simulink model "MdInOutChk"  (R2018b)
settings: Solver=FixedStepDiscrete  StartTime=0.0  StopTime=10.0  FixedStep=0.01  RelTol=1e-3
undefined symbols (not defined in the file or in its folder): MdRspLocal2
libraries: OutRspChkLib x20
(part 2 of 2)

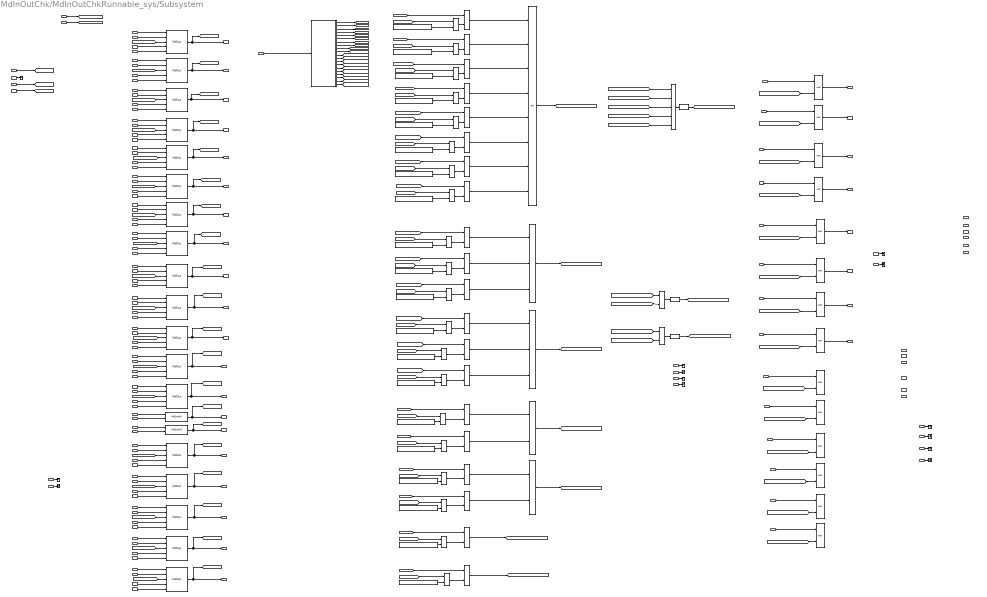
== system MdInOutChk/MdInOutChkRunnable_sys/Subsystem ==
  acsEntyMdReq_Val_read : Inport
  acsExtMdReq_Val_read : Inport  Port=2
  AllLugMdReq_Val_read : Inport  Port=3
  AllVipMdReq_Val_read : Inport  Port=4
  CommExitCond_Val_read : Inport  Port=5
  CommExitCondwithSpeed_Val_read : Inport  Port=6
  IntimacyRtMdReq_Val_read : Inport  Port=7
  INTMMdReq_Val_read : Inport  Port=8
  isAcsMdEntryDoneFailed_Val_read : Inport  Port=9
  isAcsMdEntryDoneOK_Val_read : Inport  Port=10
  isAcsMdExtDoneFailed_Val_read : Inport  Port=11
  isAcsMdExtDoneOK_Val_read : Inport  Port=12
  isINTMDoneFailed_Val_read : Inport  Port=13
  isINTMDoneOK_Val_read : Inport  Port=14
  isINTMRDoneFailed_Val_read : Inport  Port=15
  isINTMRDoneOK_Val_read : Inport  Port=16
  isLfFamlyDoneFailed_Val_read : Inport  Port=17
  isLfFamlyDoneOK_Val_read : Inport  Port=18
  isLfLugDoneFailed_Val_read : Inport  Port=19
  isLfLugDoneOK_Val_read : Inport  Port=20
  isLfLyDoneFailed_Val_read : Inport  Port=21
  isLfLyDoneOK_Val_read : Inport  Port=22
  isLfRecoveryDoneFailed_Val_read : Inport  Port=23
  isLfRecoveryDoneOK_Val_read : Inport  Port=24
  isLfVipDoneFailed_Val_read : Inport  Port=25
  isLfVipDoneOK_Val_read : Inport  Port=26
  isLgrstCloseLDoneFailed_Val_read : Inport  Port=27
  isLgrstCloseLDoneOK_Val_read : Inport  Port=28
  isLgrstCloseRDoneFailed_Val_read : Inport  Port=29
  isLgrstCloseRDoneOK_Val_read : Inport  Port=30
  isLgrstOpenLDoneFailed_Val_read : Inport  Port=31
  isLgrstOpenLDoneOK_Val_read : Inport  Port=32
  isLgrstOpenRDoneFailed_Val_read : Inport  Port=33
  isLgrstOpenRDoneOK_Val_read : Inport  Port=34
  isRfFamlyDoneFailed_Val_read : Inport  Port=35
  isRfFamlyDoneOK_Val_read : Inport  Port=36
  isRtLugDoneFailed_Val_read : Inport  Port=37
  isRtLugDoneOK_Val_read : Inport  Port=38
  isRtLyDoneFailed_Val_read : Inport  Port=39
  isRtLyDoneOK_Val_read : Inport  Port=40
  isRtRecoveryDoneFailed_Val_read : Inport  Port=41
  isRtRecoveryDoneOK_Val_read : Inport  Port=42
  isRtVipDoneFailed_Val_read : Inport  Port=43
  isRtVipDoneOK_Val_read : Inport  Port=44
  LfFamlyReq_Val_read : Inport  Port=45
  LfLyMdReq_Val_read : Inport  Port=46
  LgrstCloseLtMdReq_Val_read : Inport  Port=47
  LgrstCloseRtMdReq_Val_read : Inport  Port=48
  LgrstOpenLtMdReq_Val_read : Inport  Port=49
  LgrstOpenRtMdReq_Val_read : Inport  Port=50
  LtLugMdReq_Val_read : Inport  Port=51
  LtRcvyMdReq_Val_read : Inport  Port=52
  LtVipMdReq_Val_read : Inport  Port=53
  LugMdLtAvl_Val_read : Inport  Port=54
  LugMdRtAvl_Val_read : Inport  Port=55
  R3LMdSeatOccupied_Val_read : Inport  Port=56
  R3RMdSeatOccupied_Val_read : Inport  Port=57
  RtFamlyMdReq_Val_read : Inport  Port=58
  RtLugMdReq_Val_read : Inport  Port=59
  RtLyMdReq_Val_read : Inport  Port=60
  RtRcvyMdReq_Val_read : Inport  Port=61
  RtVipMdReq_Val_read : Inport  Port=62
  SoftIntAcsEnty_Val_read : Inport  Port=63
  SoftIntAcsExt_Val_read : Inport  Port=64
  SoftIntAllLug_Val_read : Inport  Port=65
  SoftIntAllVip_Val_read : Inport  Port=66
  SoftIntIntimacyRt_Val_read : Inport  Port=67
  SoftIntINTM_Val_read : Inport  Port=68
  SoftIntLfFamly_Val_read : Inport  Port=69
  SoftIntLfLug_Val_read : Inport  Port=70
  SoftIntLfLy_Val_read : Inport  Port=71
  SoftIntLfRcvy_Val_read : Inport  Port=72
  SoftIntLfVip_Val_read : Inport  Port=73
  SoftIntLgrstCloseLt_Val_read : Inport  Port=74
  SoftIntLgrstCloseRt_Val_read : Inport  Port=75
  SoftIntLgrstOpenLt_Val_read : Inport  Port=76
  SoftIntLgrstOpenRt_Val_read : Inport  Port=77
  SoftIntRtFamly_Val_read : Inport  Port=78
  SoftIntRtLug_Val_read : Inport  Port=79
  SoftIntRtLy_Val_read : Inport  Port=80
  SoftIntRtRcvy_Val_read : Inport  Port=81
  SoftIntRtVip_Val_read : Inport  Port=82
  StNumFlg_Is4s_read : Inport  Port=83
  StNumFlg_Is6s_read : Inport  Port=84
  StNumFlg_Is6s7s_read : Inport  Port=85
  StNumFlg_Is7s_read : Inport  Port=86
  SwIntAcsEnty_Val_read : Inport  Port=87
  SwIntAcsExt_Val_read : Inport  Port=88
  SwIntAllLug_Val_read : Inport  Port=89
  SwIntAllVip_Val_read : Inport  Port=90
  SwIntIntimacyRt_Val_read : Inport  Port=91
  SwIntINTM_Val_read : Inport  Port=92
  SwIntLfFamly_Val_read : Inport  Port=93
  SwIntLfLug_Val_read : Inport  Port=94
  SwIntLfLy_Val_read : Inport  Port=95
  SwIntLfRcvy_Val_read : Inport  Port=96
  SwIntLfVip_Val_read : Inport  Port=97
  SwIntLgrstCloseLt_Val_read : Inport  Port=98
  SwIntLgrstCloseRt_Val_read : Inport  Port=99
  SwIntLgrstOpenLt_Val_read : Inport  Port=100
  SwIntLgrstOpenRt_Val_read : Inport  Port=101
  SwIntRtFamly_Val_read : Inport  Port=102
  SwIntRtLug_Val_read : Inport  Port=103
  SwIntRtLy_Val_read : Inport  Port=104
  SwIntRtRcvy_Val_read : Inport  Port=105
  SwIntRtVip_Val_read : Inport  Port=106
  VipMdLtAvl_Val_read : Inport  Port=107
  VipMdRtAvl_Val_read : Inport  Port=108
  modestate32_Val_read : Inport  Port=109
  AND{,2..3,5..9,14..19} (14 alike) : Logic  AllPortsSameDT=off  OutDataTypeStr=boolean
  AND1 : Logic  Operator=OR  Inputs=5  AllPortsSameDT=off  OutDataTypeStr=boolean
  AND10 : Logic  Operator=OR  AllPortsSameDT=off  OutDataTypeStr=boolean
  AND11 : Logic  Operator=NOT  AllPortsSameDT=off  OutDataTypeStr=boolean
  AND12 : Logic  Operator=OR  AllPortsSameDT=off  OutDataTypeStr=boolean
  AND13 : Logic  Operator=NOT  AllPortsSameDT=off  OutDataTypeStr=boolean
  AND4 : Logic  Operator=NOT  AllPortsSameDT=off  OutDataTypeStr=boolean
  Constant{1..20} (20 alike) : Constant  Value=MdRspLocal2.MdRsp_None  OutDataTypeStr=Enum:MdRspLocal2
  Logical Operator{,1..7,9..11,14..18,21..24} (20 alike) : Logic  AllPortsSameDT=off  OutDataTypeStr=boolean
  Logical Operator12 : Logic  Operator=OR  Inputs=3  AllPortsSameDT=off  OutDataTypeStr=boolean
  Logical Operator13 : Logic  Operator=OR  Inputs=3  AllPortsSameDT=off  OutDataTypeStr=boolean
  Logical Operator19 : Logic  Operator=OR  AllPortsSameDT=off  OutDataTypeStr=boolean
  Logical Operator20 : Logic  Operator=OR  AllPortsSameDT=off  OutDataTypeStr=boolean
  Logical Operator8 : Logic  Operator=OR  Inputs=8  AllPortsSameDT=off  OutDataTypeStr=boolean
  MdOut{,1..10,12..18} (18 alike) : OutRspChkLib/MdOut  SystemSampleTime=-1
  MdOutAll : OutRspChkLib/MdOutAll  SystemSampleTime=-1
  MdOutAll1 : OutRspChkLib/MdOutAll  SystemSampleTime=-1
  ModeEnChek : Subsystem
  Relational Operator{,1..19} (20 alike) : RelationalOperator  Operator===  OutDataTypeStr=boolean  RndMeth=Simplest
  Terminator_{5,51..55,57..58,60,62..63,108..109} (13 alike) : Terminator
  acsEntyMdReqChk_Val_write : Outport
      settings: EnsureOutportIsVirtual=on
  acsExtMdReqChk_Val_write : Outport  Port=2
      settings: EnsureOutportIsVirtual=on
  AllLugMdReqChk_Val_write : Outport  Port=3
      settings: EnsureOutportIsVirtual=on
  AllVipMdReqChk_Val_write : Outport  Port=4
      settings: EnsureOutportIsVirtual=on
  EZEOutRspChk_Val_write : Outport  Port=5
      settings: EnsureOutportIsVirtual=on
  EZQOutRspChk_Val_write : Outport  Port=6
      settings: EnsureOutportIsVirtual=on
  FamlyLOutRspChk_Val_write : Outport  Port=7
      settings: EnsureOutportIsVirtual=on
  FamlyROutRspChk_Val_write : Outport  Port=8
      settings: EnsureOutportIsVirtual=on
  IntimacyRtMdReqChk_Val_write : Outport  Port=9
      settings: EnsureOutportIsVirtual=on
  INTMLOutRspChk_Val_write : Outport  Port=10
      settings: EnsureOutportIsVirtual=on
  INTMMdReqChk_Val_write : Outport  Port=11
      settings: EnsureOutportIsVirtual=on
  INTMROutRspChk_Val_write : Outport  Port=12
      settings: EnsureOutportIsVirtual=on
  LfFamlyReqChk_Val_write : Outport  Port=13
      settings: EnsureOutportIsVirtual=on
  LfLyMdReqChk_Val_write : Outport  Port=14
      settings: EnsureOutportIsVirtual=on
  LgrstCloseLtMdReqChk_Val_write : Outport  Port=15
      settings: EnsureOutportIsVirtual=on
  LgrstCloseRtMdReqChk_Val_write : Outport  Port=16
      settings: EnsureOutportIsVirtual=on
  LgrstClsLOutRspChk_Val_write : Outport  Port=17
      settings: EnsureOutportIsVirtual=on
  LgrstClsROutRspChk_Val_write : Outport  Port=18
      settings: EnsureOutportIsVirtual=on
  LgrstOpenLOutRspChk_Val_write : Outport  Port=19
      settings: EnsureOutportIsVirtual=on
  LgrstOpenLtMdReqChk_Val_write : Outport  Port=20
      settings: EnsureOutportIsVirtual=on
  LgrstOpenROutRspChk_Val_write : Outport  Port=21
      settings: EnsureOutportIsVirtual=on
  LgrstOpenRtMdReqChk_Val_write : Outport  Port=22
      settings: EnsureOutportIsVirtual=on
  LtLugMdReqChk_Val_write : Outport  Port=23
      settings: EnsureOutportIsVirtual=on
  LtRcvyMdReqChk_Val_write : Outport  Port=24
      settings: EnsureOutportIsVirtual=on
  LtVipMdReqChk_Val_write : Outport  Port=25
      settings: EnsureOutportIsVirtual=on
  LugAllOutRspChk_Val_write : Outport  Port=26
      settings: EnsureOutportIsVirtual=on
  LugLOutRspChk_Val_write : Outport  Port=27
      settings: EnsureOutportIsVirtual=on
  LugROutRspChk_Val_write : Outport  Port=28
      settings: EnsureOutportIsVirtual=on
  LyLOutRspChk_Val_write : Outport  Port=29
      settings: EnsureOutportIsVirtual=on
  LyROutRspChk_Val_write : Outport  Port=30
      settings: EnsureOutportIsVirtual=on
  RcvyLOutRspChk_Val_write : Outport  Port=31
      settings: EnsureOutportIsVirtual=on
  RcvyROutRspChk_Val_write : Outport  Port=32
      settings: EnsureOutportIsVirtual=on
  RtFamlyMdReqChk_Val_write : Outport  Port=33
      settings: EnsureOutportIsVirtual=on
  RtLugMdReqChk_Val_write : Outport  Port=34
      settings: EnsureOutportIsVirtual=on
  RtLyMdReqChk_Val_write : Outport  Port=35
      settings: EnsureOutportIsVirtual=on
  RtRcvyMdReqChk_Val_write : Outport  Port=36
      settings: EnsureOutportIsVirtual=on
  RtVipMdReqChk_Val_write : Outport  Port=37
      settings: EnsureOutportIsVirtual=on
  VIPALLOutRspChk_Val_write : Outport  Port=38
      settings: EnsureOutportIsVirtual=on
  VIPLOutRspChk_Val_write : Outport  Port=39
      settings: EnsureOutportIsVirtual=on
  VIPROutRspChk_Val_write : Outport  Port=40
      settings: EnsureOutportIsVirtual=on
  wires:
  R3RMdSeatOccupied_Val_read/1 -> Terminator_58/1
  isINTMRDoneOK_Val_read/1 -> MdOut3/2
  LtRcvyMdReq_Val_read/1 -> Terminator_52/1
  LgrstCloseRtMdReq_Val_read/1 -> AND18/1
  CommExitCond_Val_read/1 -> [CommExitCond]
  isINTMRDoneFailed_Val_read/1 -> MdOut3/1
  isAcsMdEntryDoneOK_Val_read/1 -> MdOut/2
  LugMdLtAvl_Val_read/1 -> Terminator_54/1
  isLfFamlyDoneFailed_Val_read/1 -> MdOut4/1
  isRfFamlyDoneOK_Val_read/1 -> MdOut5/2
  VipMdRtAvl_Val_read/1 -> Terminator_109/1
  LfLyMdReq_Val_read/1 -> AND14/1
  isAcsMdExtDoneOK_Val_read/1 -> MdOut1/2
  SwIntLfFamly_Val_read/1 -> MdOut4/4
  isINTMDoneOK_Val_read/1 -> MdOut2/2
  isAcsMdExtDoneFailed_Val_read/1 -> MdOut1/1
  SoftIntAcsEnty_Val_read/1 -> MdOut/5
  StNumFlg_Is4s_read/1 -> [Is4s]
  CommExitCondwithSpeed_Val_read/1 -> [CommExitCondwithSpeed]
  isRfFamlyDoneFailed_Val_read/1 -> MdOut5/1
  isINTMDoneFailed_Val_read/1 -> MdOut2/1
  isAcsMdEntryDoneFailed_Val_read/1 -> MdOut/1
  LgrstOpenLtMdReq_Val_read/1 -> AND16/1
  isLfLugDoneOK_Val_read/1 -> MdOut6/2
  LugMdRtAvl_Val_read/1 -> Terminator_55/1
  isLfFamlyDoneOK_Val_read/1 -> MdOut4/2
  RtLugMdReq_Val_read/1 -> Terminator_60/1
  RtLyMdReq_Val_read/1 -> AND17/1
  isLgrstCloseLDoneOK_Val_read/1 -> MdOut8/2
  LtVipMdReq_Val_read/1 -> Terminator_53/1
  RtVipMdReq_Val_read/1 -> Terminator_63/1
  SwIntLfLug_Val_read/1 -> MdOut6/4
  R3LMdSeatOccupied_Val_read/1 -> Terminator_57/1
  SoftIntLgrstOpenLt_Val_read/1 -> MdOut10/5
  StNumFlg_Is6s_read/1 -> [Is6s]
  StNumFlg_Is7s_read/1 -> [Is7s]
  LtLugMdReq_Val_read/1 -> Terminator_51/1
  isLfLugDoneFailed_Val_read/1 -> MdOut6/1
  isRtVipDoneOK_Val_read/1 -> MdOut18/2
  VipMdLtAvl_Val_read/1 -> Terminator_108/1
  RtRcvyMdReq_Val_read/1 -> Terminator_62/1
  [CommExitCondwithSpeed] -> MdOut/3
  SoftIntAcsExt_Val_read/1 -> MdOut1/5
  SoftIntINTM_Val_read/1 -> MdOut2/5
  SoftIntIntimacyRt_Val_read/1 -> MdOut3/5
  SoftIntLfFamly_Val_read/1 -> MdOut4/5
  SoftIntRtFamly_Val_read/1 -> MdOut5/5
  isLfLyDoneFailed_Val_read/1 -> MdOut7/1
  isLfLyDoneOK_Val_read/1 -> MdOut7/2
  isLgrstCloseLDoneFailed_Val_read/1 -> MdOut8/1
  SoftIntLgrstCloseLt_Val_read/1 -> MdOut8/5
  SoftIntLfLy_Val_read/1 -> MdOut7/5
  isLgrstCloseRDoneFailed_Val_read/1 -> MdOut9/1
  isLgrstCloseRDoneOK_Val_read/1 -> MdOut9/2
  isLgrstOpenLDoneFailed_Val_read/1 -> MdOut10/1
  isLgrstOpenRDoneFailed_Val_read/1 -> MdOut12/1
  isLgrstOpenRDoneOK_Val_read/1 -> MdOut12/2
  isRtLugDoneFailed_Val_read/1 -> MdOut13/1
  isRtLugDoneOK_Val_read/1 -> MdOut13/2
  isRtLyDoneFailed_Val_read/1 -> MdOut14/1
  isRtLyDoneOK_Val_read/1 -> MdOut14/2
  isLfRecoveryDoneFailed_Val_read/1 -> MdOut15/1
  isLfRecoveryDoneOK_Val_read/1 -> MdOut15/2
  isLfVipDoneFailed_Val_read/1 -> MdOut16/1
  isLfVipDoneOK_Val_read/1 -> MdOut16/2
  isRtRecoveryDoneFailed_Val_read/1 -> MdOut17/1
  isRtRecoveryDoneOK_Val_read/1 -> MdOut17/2
  isRtVipDoneFailed_Val_read/1 -> MdOut18/1
  SoftIntLgrstCloseRt_Val_read/1 -> MdOut9/5
  SoftIntLfLug_Val_read/1 -> MdOut6/5
  SoftIntRtLug_Val_read/1 -> MdOut13/5
  SoftIntRtLy_Val_read/1 -> MdOut14/5
  SoftIntLfRcvy_Val_read/1 -> MdOut15/5
  SoftIntRtRcvy_Val_read/1 -> MdOut17/5
  SoftIntRtVip_Val_read/1 -> MdOut18/5
  SoftIntLfVip_Val_read/1 -> MdOut16/5
  SwIntAcsEnty_Val_read/1 -> MdOut/4
  SwIntAcsExt_Val_read/1 -> MdOut1/4
  [CommExitCondwithSpeed] -> MdOut1/3
  SwIntINTM_Val_read/1 -> MdOut2/4
  [CommExitCond] -> MdOut2/3
  [CommExitCond] -> MdOut3/3
  SwIntIntimacyRt_Val_read/1 -> MdOut3/4
  [CommExitCond] -> MdOut4/3
  [CommExitCond] -> MdOut5/3
  SwIntRtRcvy_Val_read/1 -> MdOut17/4
  SwIntRtLy_Val_read/1 -> MdOut14/4
  SwIntRtLug_Val_read/1 -> MdOut13/4
  SwIntLgrstOpenRt_Val_read/1 -> MdOut12/4
  SwIntLgrstOpenLt_Val_read/1 -> MdOut10/4
  SwIntLgrstCloseRt_Val_read/1 -> MdOut9/4
  SwIntLgrstCloseLt_Val_read/1 -> MdOut8/4
  SwIntLfLy_Val_read/1 -> MdOut7/4
  SwIntRtFamly_Val_read/1 -> MdOut5/4
  [CommExitCondwithSpeed] -> MdOut6/3
  [CommExitCond] -> MdOut7/3
  [CommExitCond] -> MdOut8/3
  [CommExitCond] -> MdOut9/3
  [CommExitCond] -> MdOut10/3
  isLgrstOpenLDoneOK_Val_read/1 -> MdOut10/2
  SoftIntLgrstOpenRt_Val_read/1 -> MdOut12/5
  [CommExitCond] -> MdOut12/3
  [CommExitCondwithSpeed] -> MdOut13/3
  [CommExitCond] -> MdOut14/3
  [CommExitCond] -> MdOut15/3
  SwIntLfRcvy_Val_read/1 -> MdOut15/4
  SwIntLfVip_Val_read/1 -> MdOut16/4
  [CommExitCond] -> MdOut16/3
  [CommExitCond] -> MdOut17/3
  [CommExitCond] -> MdOut18/3
  SwIntRtVip_Val_read/1 -> MdOut18/4
  SoftIntAllVip_Val_read/1 -> MdOutAll/2
  SwIntAllVip_Val_read/1 -> MdOutAll/1
  SoftIntAllLug_Val_read/1 -> MdOutAll1/2
  SwIntAllLug_Val_read/1 -> MdOutAll1/1
  MdOut/1 -> [EZEOutRspChk], EZEOutRspChk_Val_write/1
  MdOut1/1 -> [EZQOutRspChk], EZQOutRspChk_Val_write/1
  MdOut2/1 -> [INTMLOutRspChk], INTMLOutRspChk_Val_write/1
  MdOut3/1 -> [INTMROutRspChk], INTMROutRspChk_Val_write/1
  MdOut4/1 -> [FamlyLOutRspChk], FamlyLOutRspChk_Val_write/1
  MdOut5/1 -> [FamlyROutRspChk], FamlyROutRspChk_Val_write/1
  MdOut6/1 -> [LugLOutRspChk], LugLOutRspChk_Val_write/1
  MdOut13/1 -> [LugROutRspChk], LugROutRspChk_Val_write/1
  MdOut7/1 -> [LyLOutRspChk], LyLOutRspChk_Val_write/1
  MdOut8/1 -> [LgrstClsLOutRspChk], LgrstClsLOutRspChk_Val_write/1
  MdOut10/1 -> [LgrstOpenLOutRspChk], LgrstOpenLOutRspChk_Val_write/1
  MdOut12/1 -> [LgrstOpenROutRspChk], LgrstOpenROutRspChk_Val_write/1
  MdOut9/1 -> [LgrstClsROutRspChk], LgrstClsROutRspChk_Val_write/1
  MdOutAll/1 -> [VIPALLOutRspChk], VIPALLOutRspChk_Val_write/1
  MdOut15/1 -> [RcvyLOutRspChk], RcvyLOutRspChk_Val_write/1
  MdOut16/1 -> [VIPLOutRspChk], VIPLOutRspChk_Val_write/1
  MdOut17/1 -> [RcvyROutRspChk], RcvyROutRspChk_Val_write/1
  MdOut18/1 -> [VIPROutRspChk], VIPROutRspChk_Val_write/1
  MdOutAll1/1 -> [LugAllOutRspChk], LugAllOutRspChk_Val_write/1
  MdOut14/1 -> [LyROutRspChk], LyROutRspChk_Val_write/1
  StNumFlg_Is6s7s_read/1 -> Terminator_5/1
  [EZEOutRspChk] -> Relational Operator/1
  ModeEnChek/11(INTM_En) -> [INTM_En]
  ModeEnChek/18(LgrstOpenR_En) -> [LgrstOpenR_En]
  ModeEnChek/10(LugAll_En) -> [LugAll_En]
  ModeEnChek/9(VIPAll_En) -> [VIPAll_En]
  ModeEnChek/14(LyL_En) -> [LyL_En]
  ModeEnChek/19(LgrstCloseR_En) -> [LgrstCloseR_En]
  ModeEnChek/12(FAMLY_L_En) -> [FAMLY_L_En]
  ModeEnChek/3(Recovery_L_En) -> [Recovery_L]
  ModeEnChek/4(Recovery_R_En) -> [Recovery_R]
  ModeEnChek/8(EZQ_En) -> [EZQ_En]
  ModeEnChek/6(Lug_R_En) -> [Lug_R]
  ModeEnChek/5(Lug_L_En) -> [Lug_L]
  ModeEnChek/7(EZE_En) -> [EZE_En]
  ModeEnChek/16(LgrstOpenL_En) -> [LgrstOpenL_En]
  ModeEnChek/13(FAMLY_R_En) -> [FAMLY_R_En]
  ModeEnChek/15(LyR_En) -> [LyR_En]
  ModeEnChek/20(INTMR_En) -> [INTMR_En]
  ModeEnChek/2(VIP_R_En) -> [VIP_R]
  ModeEnChek/17(LgrstCloseL_En) -> [LgrstCloseL_En]
  ModeEnChek/1(VIP_L_En) -> [VIP_L]
  modestate32_Val_read/1 -> ModeEnChek/1(modestate32)
  [EZE_En] -> Logical Operator/1
  Relational Operator/1 -> Logical Operator/2
  Constant1/1 -> Relational Operator/2
  [EZQ_En] -> Logical Operator1/1
  Relational Operator1/1 -> Logical Operator1/2
  [EZQOutRspChk] -> Relational Operator1/1
  Constant2/1 -> Relational Operator1/2
  [VIPAll_En] -> Logical Operator2/1
  Relational Operator2/1 -> Logical Operator2/2
  [VIPALLOutRspChk] -> Relational Operator2/1
  Constant3/1 -> Relational Operator2/2
  [LugAll_En] -> Logical Operator3/1
  Relational Operator3/1 -> Logical Operator3/2
  [LugAllOutRspChk] -> Relational Operator3/1
  Constant4/1 -> Relational Operator3/2
  [INTM_En] -> Logical Operator4/1
  Relational Operator4/1 -> Logical Operator4/2
  [INTMLOutRspChk] -> Relational Operator4/1
  Constant5/1 -> Relational Operator4/2
  Relational Operator5/1 -> Logical Operator5/2
  [INTMR_En] -> Logical Operator5/1
  [INTMROutRspChk] -> Relational Operator5/1
  Constant6/1 -> Relational Operator5/2
  [FAMLY_L_En] -> Logical Operator6/1
  Relational Operator6/1 -> Logical Operator6/2
  [FamlyLOutRspChk] -> Relational Operator6/1
  Constant7/1 -> Relational Operator6/2
  [FAMLY_R_En] -> Logical Operator7/1
  Relational Operator7/1 -> Logical Operator7/2
  [FamlyROutRspChk] -> Relational Operator7/1
  Constant8/1 -> Relational Operator7/2
  Logical Operator/1 -> Logical Operator8/1
  Logical Operator1/1 -> Logical Operator8/2
  Logical Operator2/1 -> Logical Operator8/3
  Logical Operator3/1 -> Logical Operator8/4
  Logical Operator4/1 -> Logical Operator8/5
  Logical Operator5/1 -> Logical Operator8/6
  Logical Operator6/1 -> Logical Operator8/7
  Logical Operator7/1 -> Logical Operator8/8
  Logical Operator8/1 -> [MaskAllReq6s7s]
  [LyL_En] -> Logical Operator9/1
  Relational Operator8/1 -> Logical Operator9/2
  Constant9/1 -> Relational Operator8/2
  [LyLOutRspChk] -> Relational Operator8/1
  Relational Operator9/1 -> Logical Operator10/2
  [LgrstOpenL_En] -> Logical Operator10/1
  [LgrstOpenLOutRspChk] -> Relational Operator9/1
  Constant10/1 -> Relational Operator9/2
  [LgrstCloseL_En] -> Logical Operator11/1
  Relational Operator10/1 -> Logical Operator11/2
  Constant11/1 -> Relational Operator10/2
  [LgrstClsLOutRspChk] -> Relational Operator10/1
  Logical Operator9/1 -> Logical Operator12/1
  Logical Operator10/1 -> Logical Operator12/2
  Logical Operator11/1 -> Logical Operator12/3
  Logical Operator12/1 -> [MaskLReq4s]
  Logical Operator14/1 -> Logical Operator13/1
  Logical Operator15/1 -> Logical Operator13/2
  Logical Operator16/1 -> Logical Operator13/3
  Relational Operator11/1 -> Logical Operator14/2
  Relational Operator12/1 -> Logical Operator15/2
  Relational Operator13/1 -> Logical Operator16/2
  [LyR_En] -> Logical Operator14/1
  [LgrstCloseR_En] -> Logical Operator16/1
  [LyROutRspChk] -> Relational Operator11/1
  [LgrstOpenROutRspChk] -> Relational Operator12/1
  [LgrstOpenR_En] -> Logical Operator15/1
  [LgrstClsROutRspChk] -> Relational Operator13/1
  Constant12/1 -> Relational Operator11/2
  Constant13/1 -> Relational Operator12/2
  Constant14/1 -> Relational Operator13/2
  Logical Operator13/1 -> [MaskRReq4s]
  Logical Operator17/1 -> Logical Operator19/1
  Logical Operator18/1 -> Logical Operator19/2
  Relational Operator14/1 -> Logical Operator17/2
  Relational Operator15/1 -> Logical Operator18/2
  [RcvyLOutRspChk] -> Relational Operator14/1
  [VIPLOutRspChk] -> Relational Operator15/1
  Constant15/1 -> Relational Operator14/2
  Constant16/1 -> Relational Operator15/2
  [Recovery_L] -> Logical Operator17/1
  [VIP_L] -> Logical Operator18/1
  Logical Operator22/1 -> Logical Operator20/2
  Logical Operator21/1 -> Logical Operator20/1
  Relational Operator16/1 -> Logical Operator21/2
  Relational Operator17/1 -> Logical Operator22/2
  [RcvyROutRspChk] -> Relational Operator16/1
  [VIPROutRspChk] -> Relational Operator17/1
  Constant17/1 -> Relational Operator16/2
  Constant18/1 -> Relational Operator17/2
  [Recovery_R] -> Logical Operator21/1
  [VIP_R] -> Logical Operator22/1
  Logical Operator19/1 -> [MaskLReq6s7s4s]
  Logical Operator20/1 -> [MaskRReq6s7s4s]
  [Lug_L] -> Logical Operator23/1
  Relational Operator18/1 -> Logical Operator23/2
  Constant19/1 -> Relational Operator18/2
  Relational Operator19/1 -> Logical Operator24/2
  Constant20/1 -> Relational Operator19/2
  [Lug_R] -> Logical Operator24/1
  [LugLOutRspChk] -> Relational Operator18/1
  [LugROutRspChk] -> Relational Operator19/1
  Logical Operator23/1 -> [MaskReqFrmLugL]
  Logical Operator24/1 -> [MaskReqFromLugR]
  AND/1 -> acsEntyMdReqChk_Val_write/1
  [MaskAllReq6s7s] -> AND1/1
  [MaskLReq6s7s4s] -> AND1/2
  [MaskRReq6s7s4s] -> AND1/3
  [MaskReqFrmLugL] -> AND1/4
  [MaskReqFromLugR] -> AND1/5
  AND1/1 -> AND4/1
  AND2/1 -> acsExtMdReqChk_Val_write/1
  [NotMaskAllMd] -> AND2/2
  acsExtMdReq_Val_read/1 -> AND2/1
  acsEntyMdReq_Val_read/1 -> AND/1
  [NotMaskAllMd] -> AND/2
  AND4/1 -> [NotMaskAllMd]
  AND3/1 -> AllLugMdReqChk_Val_write/1
  [NotMaskAllMd] -> AND3/2
  AND5/1 -> AllVipMdReqChk_Val_write/1
  [NotMaskAllMd] -> AND5/2
  AND6/1 -> IntimacyRtMdReqChk_Val_write/1
  AND7/1 -> INTMMdReqChk_Val_write/1
  AND8/1 -> LfFamlyReqChk_Val_write/1
  AND9/1 -> RtFamlyMdReqChk_Val_write/1
  IntimacyRtMdReq_Val_read/1 -> AND6/1
  INTMMdReq_Val_read/1 -> AND7/1
  LfFamlyReq_Val_read/1 -> AND8/1
  RtFamlyMdReq_Val_read/1 -> AND9/1
  AllVipMdReq_Val_read/1 -> AND5/1
  AllLugMdReq_Val_read/1 -> AND3/1
  [NotMaskAllMd] -> AND6/2
  [NotMaskAllMd] -> AND7/2
  [NotMaskAllMd] -> AND8/2
  [NotMaskAllMd] -> AND9/2
  AND10/1 -> AND11/1
  [MaskLReq4s] -> AND10/1
  [MaskLReq6s7s4s] -> AND10/2
  [MaskRReq4s] -> AND12/1
  [MaskRReq6s7s4s] -> AND12/2
  AND12/1 -> AND13/1
  AND11/1 -> [NotMask4sLMd]
  AND13/1 -> [NotMask4sRMd]
  [NotMask4sLMd] -> AND14/2
  [NotMask4sLMd] -> AND15/2
  LgrstCloseLtMdReq_Val_read/1 -> AND15/1
  [NotMask4sLMd] -> AND16/2
  LgrstOpenRtMdReq_Val_read/1 -> AND19/1
  [NotMask4sRMd] -> AND17/2
  [NotMask4sRMd] -> AND18/2
  [NotMask4sRMd] -> AND19/2

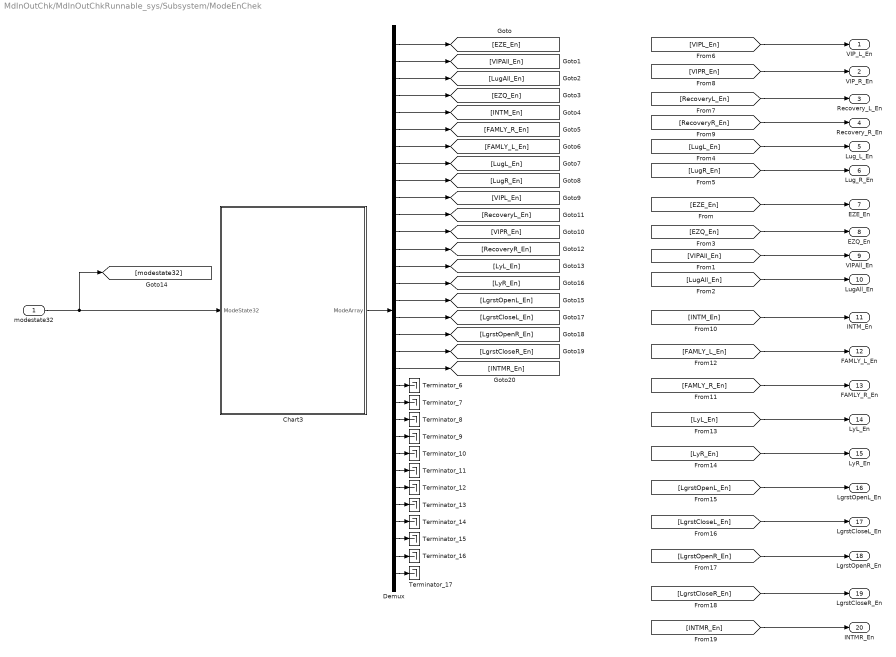
== system MdInOutChk/MdInOutChkRunnable_sys/Subsystem/ModeEnChek ==
  modestate32 : Inport
  Chart3 : Stateflow chart  TreatAsAtomicUnit=on
  Demux : Demux  Outputs=32
  Terminator_{6..17} (12 alike) : Terminator
  VIP_L_En : Outport
  VIP_R_En : Outport  Port=2
  Recovery_L_En : Outport  Port=3
  Recovery_R_En : Outport  Port=4
  Lug_L_En : Outport  Port=5
  Lug_R_En : Outport  Port=6
  EZE_En : Outport  Port=7
  EZQ_En : Outport  Port=8
  VIPAll_En : Outport  Port=9
  LugAll_En : Outport  Port=10
  INTM_En : Outport  Port=11
  FAMLY_L_En : Outport  Port=12
  FAMLY_R_En : Outport  Port=13
  LyL_En : Outport  Port=14
  LyR_En : Outport  Port=15
  LgrstOpenL_En : Outport  Port=16
  LgrstCloseL_En : Outport  Port=17
  LgrstOpenR_En : Outport  Port=18
  LgrstCloseR_En : Outport  Port=19
  INTMR_En : Outport  Port=20
  wires:
  Chart3/1(ModeArray) -> Demux/1
  Demux/1 -> [EZE_En]
  Demux/2 -> [VIPAll_En]
  Demux/3 -> [LugAll_En]
  Demux/4 -> [EZQ_En]
  Demux/5 -> [INTM_En]
  Demux/6 -> [FAMLY_R_En]
  Demux/7 -> [FAMLY_L_En]
  Demux/8 -> [LugL_En]
  Demux/9 -> [LugR_En]
  Demux/10 -> [VIPL_En]
  Demux/12 -> [VIPR_En]
  Demux/11 -> [RecoveryL_En]
  Demux/13 -> [RecoveryR_En]
  Demux/14 -> [LyL_En]
  Demux/15 -> [LyR_En]
  modestate32/1 -> [modestate32], Chart3/1(ModeState32)
  [EZE_En] -> EZE_En/1
  [EZQ_En] -> EZQ_En/1
  [VIPL_En] -> VIP_L_En/1
  [VIPR_En] -> VIP_R_En/1
  [RecoveryL_En] -> Recovery_L_En/1
  [RecoveryR_En] -> Recovery_R_En/1
  [LugL_En] -> Lug_L_En/1
  [LugR_En] -> Lug_R_En/1
  [VIPAll_En] -> VIPAll_En/1
  [LugAll_En] -> LugAll_En/1
  Demux/16 -> [LgrstOpenL_En]
  Demux/17 -> [LgrstCloseL_En]
  Demux/18 -> [LgrstOpenR_En]
  Demux/19 -> [LgrstCloseR_En]
  Demux/20 -> [INTMR_En]
  Demux/21 -> Terminator_6/1
  Demux/22 -> Terminator_7/1
  Demux/23 -> Terminator_8/1
  Demux/24 -> Terminator_9/1
  Demux/25 -> Terminator_10/1
  Demux/26 -> Terminator_11/1
  Demux/27 -> Terminator_12/1
  Demux/28 -> Terminator_13/1
  Demux/29 -> Terminator_14/1
  Demux/30 -> Terminator_15/1
  Demux/31 -> Terminator_16/1
  Demux/32 -> Terminator_17/1
  [INTM_En] -> INTM_En/1
  [FAMLY_L_En] -> FAMLY_L_En/1
  [FAMLY_R_En] -> FAMLY_R_En/1
  [LyR_En] -> LyR_En/1
  [LyL_En] -> LyL_En/1
  [LgrstOpenL_En] -> LgrstOpenL_En/1
  [LgrstCloseL_En] -> LgrstCloseL_En/1
  [LgrstOpenR_En] -> LgrstOpenR_En/1
  [LgrstCloseR_En] -> LgrstCloseR_En/1
  [INTMR_En] -> INTMR_En/1

== stateflow chart MdInOutChk/MdInOutChkRunnable_sys/Subsystem/ModeEnChek/Chart3 ==
  (default) -> (junction 3)
  (junction 3) -> (junction 9) : {i = 0;}
  (junction 9) -> (junction 4) [order 1] : [i < 32]
  (junction 4) -> (junction 1) : {
      | temp_var = 0x00000001 & (ModeState32>>i);
      | ModeArray[i] =boolean(temp_var);
      | }
  (junction 1) -> (junction 9) : {i++;}
  (junction 9) -> (junction 5) [order 2]
  data: temp_var local uint32; ModeState32 input uint32; ModeArray output boolean size=32; i local uint8
